simulink model "basic_robust"  (R2020a)
settings: Solver=VariableStepAuto  StartTime=0.0  StopTime=10.0  RelTol=1e-3
settings Model: Creator=ripme  LastModifiedBy=ripme
settings SolverCC: ZeroCrossAlgorithm=Adaptive
settings DebuggingCC: IgnoredZcDiagnostic=none

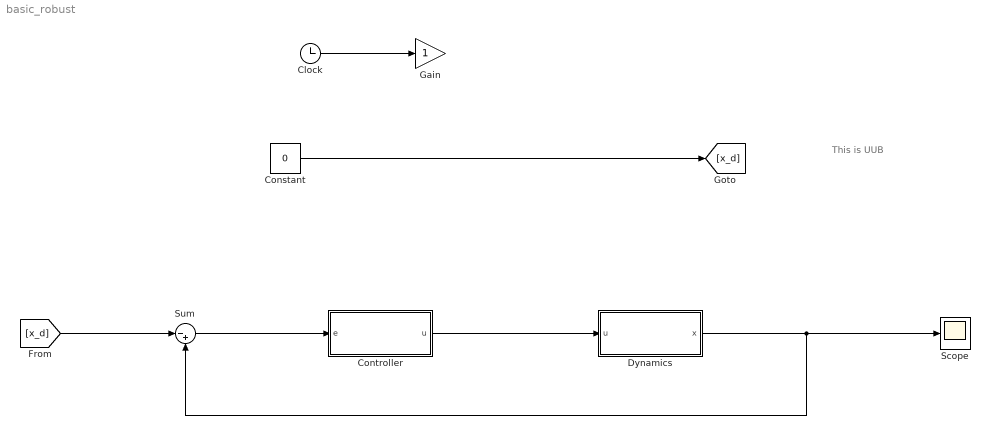
== system basic_robust ==
  note: This is UUB
  Clock : Clock
  Constant : Constant  Value=0
  Controller : Subsystem
  Dynamics : Subsystem
  Gain : Gain
  Scope : Scope
  Sum : Sum  Inputs=|-+
  wires:
  Controller/1(u) -> Dynamics/1(u)
  [x_d] -> Sum/1
  Clock/1 -> Gain/1
  Constant/1 -> [x_d]
  Sum/1 -> Controller/1(e)
  Dynamics/1(x) -> Sum/2, Scope/1

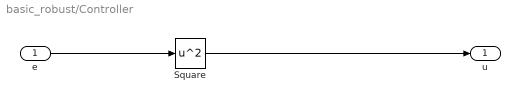
== system basic_robust/Controller ==
  e : Inport
  Square : Math  Operator=square  SaturateOnIntegerOverflow=on
  u : Outport
  wires:
  e/1 -> Square/1
  Square/1 -> u/1

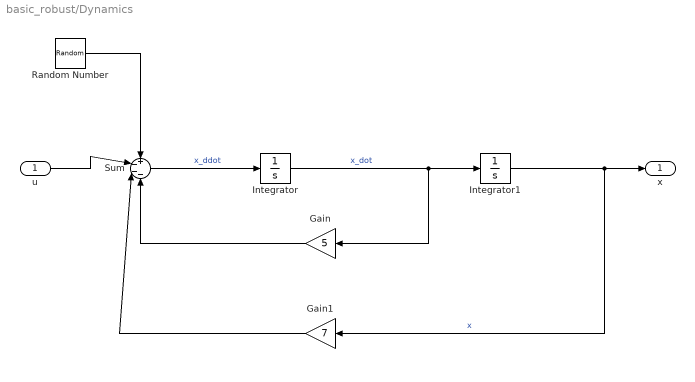
== system basic_robust/Dynamics ==
  u : Inport
  Gain : Gain  Gain=5
  Gain1 : Gain  Gain=7
  Integrator : Integrator  InitialCondition=20
  Integrator1 : Integrator  InitialCondition=20
  Random Number : RandomNumber  SampleTime=0.1
  Sum : Sum  Inputs=+---
  x : Outport
  wires:
  Sum/1 -> Integrator/1  "x_ddot"
  Integrator/1 -> Gain/1, Integrator1/1  "x_dot"
  Integrator1/1 -> Gain1/1, x/1  "x"
  u/1 -> Sum/2
  Gain/1 -> Sum/4
  Gain1/1 -> Sum/3
  Random Number/1 -> Sum/1
